simulink model "Controllori"  (R2020b)
settings: Solver=VariableStepAuto  StartTime=0.0  StopTime=6  RelTol=1e-3
values from neighbouring files (symbols this model uses):
  A_num = eval(A)    [eq_non_linear.m]
  B_num = eval(B)    [eq_non_linear.m]
  C_num = eval(C)    [eq_non_linear.m]
  D_num = eval(D)    [eq_non_linear.m]
  G0_fb_lqr_R = dcgain(reg_fb_lqr_R)    [controlloLQR.m]    (also in lqr_params.m)
  G0_fb_lqr_Y = dcgain(reg_fb_lqr_Y)    [controlloLQR.m]    (also in lqr_params.m)
  G0_fb_lqr_z = dcgain(reg_fb_lqr_z)    [controlloLQR.m]    (also in lqr_params.m)
  G0_fb_R = dcgain(reg_fb_R)    [controllo.m]
  G0_fb_Y = dcgain(reg_fb_Y)    [controllo.m]
  G0_fb_z = dcgain(reg_fb_z)    [controllo.m]
  reg_dir_lqr_R = ss(A_R-B_R*K_lqr_R-L_lqr_R*C_R,L_lqr_R,K_lqr_R,0)    [controlloLQR.m]    (also in lqr_params.m)
  reg_dir_lqr_Y = ss(A_Y-B_Y*K_lqr_Y-L_lqr_Y*C_Y,L_lqr_Y,K_lqr_Y,0)    [controlloLQR.m]    (also in lqr_params.m)
  reg_dir_lqr_z = ss(A_z-B_z*K_lqr_z-L_lqr_z*C_z,L_lqr_z,K_lqr_z,0)    [controlloLQR.m]    (also in lqr_params.m)
  reg_dir_R = ss(A_R-B_R*K_R-L_R*C_R,L_R,K_R,0)    [controllo.m]
  reg_dir_Y = ss(A_Y-B_Y*K_Y-L_Y*C_Y,L_Y,K_Y,0)    [controllo.m]
  reg_dir_z = ss(A_z-B_z*K_z-L_z*C_z,L_z,K_z,0)    [controllo.m]
  reg_fb_lqr_R = ss(A_R-B_R*K_lqr_R-L_lqr_R*C_R,-L_lqr_R,-K_lqr_R,0)    [controlloLQR.m]    (also in lqr_params.m)
  reg_fb_lqr_Y = ss(A_Y-B_Y*K_lqr_Y-L_lqr_Y*C_Y,-L_lqr_Y,-K_lqr_Y,0)    [controlloLQR.m]    (also in lqr_params.m)
  reg_fb_lqr_z = ss(A_z-B_z*K_lqr_z-L_lqr_z*C_z,-L_lqr_z,-K_lqr_z,0)    [controlloLQR.m]    (also in lqr_params.m)
  reg_fb_R = ss(A_R-B_R*K_R-L_R*C_R,-L_R,-K_R,0)    [controllo.m]
  reg_fb_Y = ss(A_Y-B_Y*K_Y-L_Y*C_Y,-L_Y,-K_Y,0)    [controllo.m]
  reg_fb_z = ss(A_z-B_z*K_z-L_z*C_z,-L_z,-K_z,0)    [controllo.m]
undefined symbols (not defined in the file or in its folder): A_PID, B_PID, C_PID, D_PID
libraries: pid_lib x8, simulink x1
settings Model: Creator=Tommaso  LastModifiedBy=Tommaso

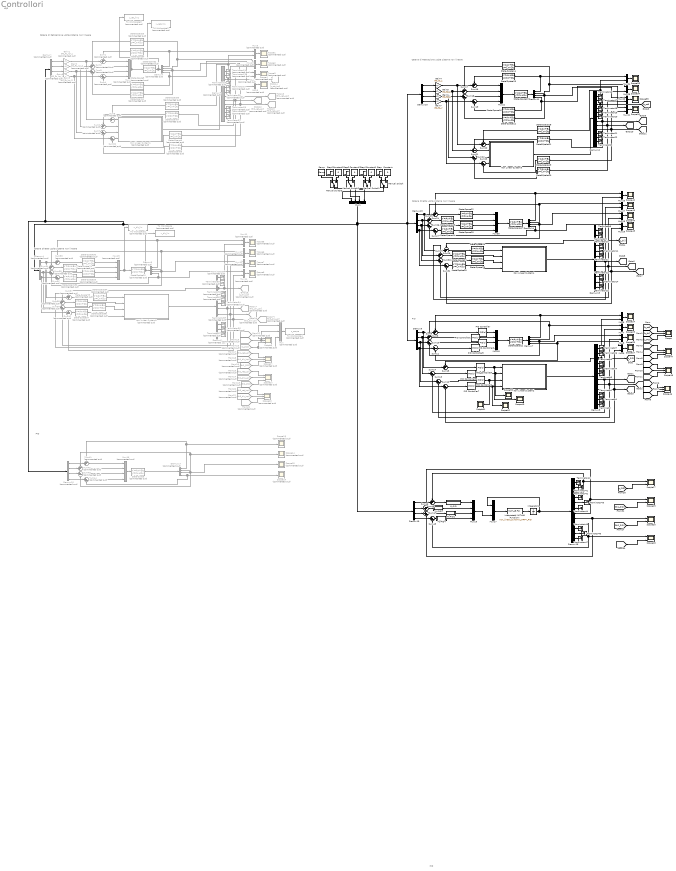
== system Controllori ==
  note: PID
  note: LQR
  note: PID
  note: Catena di Retroazione uscite sistema non lineare
  note: Catena Diretta uscita sistema non lineare
  note: Catena di Retroazione uscite sistema non lineare
  note: Catena Diretta uscita sistema non lineare
  note: PID
  Constant{,1..3} (4 alike) : Constant  Value=0
  Demux{1..2,4..5,16..17} (6 alike) : Demux  Commented=on
  Demux{7,9..11,13..14,19} (7 alike) : Demux
  Demux{8,12,15,18} (4 alike) : Demux  Outputs=12
  Demux3 : Demux  Commented=on  Outputs=12
  Demux6 : Demux  Commented=on  Outputs=12
  From12 : From  Commented=on  GotoTag=z_ret_Lqr
  From13 : From  Commented=on  GotoTag=z_dir_Lqr
  From14 : From  Commented=on  GotoTag=th2_dir_Lqr
  From15 : From  Commented=on  GotoTag=th2_PID
  From16 : From  Commented=on  GotoTag=z_PID
  From17 : From  Commented=on  GotoTag=th1_ret_Lqr
  From18 : From  Commented=on  GotoTag=th1_dir_Lqr
  From19 : From  Commented=on  GotoTag=th1_PID
  From20 : From  Commented=on  GotoTag=th3_ret_Lqr
  From21 : From  Commented=on  GotoTag=th3_dir_Lqr
  From22 : From  Commented=on  GotoTag=th3_PID
  From23 : From  Commented=on  GotoTag=th2_ret_Lqr
  Gain1 : Gain  Commented=on  Gain=G0_fb_lqr_z
  Gain2 : Gain  Commented=on  Gain=G0_fb_lqr_R
  Gain3 : Gain  Commented=on  Gain=G0_fb_lqr_R
  Gain4 : Gain  Gain=G0_fb_z
  Gain5 : Gain  Gain=G0_fb_R
  Gain6 : Gain  Gain=G0_fb_R
  Gain7 : Gain  Gain=G0_fb_Y
  Gain8 : Gain  Commented=on  Gain=G0_fb_lqr_Y
  Goto12 : Goto  Commented=on  GotoTag=th2_ret_Lqr
  Goto13 : Goto  Commented=on  GotoTag=th3_ret_Lqr
  Goto14 : Goto  Commented=on  GotoTag=z_ret_Lqr
  Goto15 : Goto  Commented=on  GotoTag=th1_ret_Lqr
  Goto16 : Goto  Commented=on  GotoTag=z_dir_Lqr
  Goto17 : Goto  Commented=on  GotoTag=th1_dir_Lqr
  Goto18 : Goto  Commented=on  GotoTag=th2_dir_Lqr
  Goto19 : Goto  Commented=on  GotoTag=th3_dir_Lqr
  Integrator1 : Integrator  InitialCondition=[0,0,0,0,0,0,0,0,0,0,0,0]
  Interpreted MATLAB Function1 : MATLABFcn  MATLABFcn=non_linear_dynamic_HRPY_PID
  Manual Switch{,1..3} (4 alike) : ManualSwitch
  Mux : Mux  Commented=on  Inputs=3
  Mux{1,18..19,22,30} (5 alike) : Mux
  Mux{2..3,5,10..14} (8 alike) : Mux  Commented=on  Inputs=2
  Mux15 : Mux  Commented=on
  Mux16 : Mux  Commented=on
  Mux{6..9,17,20..21,24..29} (13 alike) : Mux  Inputs=2
  Mux4 : Mux  Commented=on
  MyPID : Subsystem
  MyPID1 : Subsystem
  MyPID2 : Subsystem
  MyPID4 : Subsystem
  Non Linear System1 : Subsystem  Commented=on
  Non Linear System2 : Subsystem
  Non Linear System3 : Subsystem
  Non Linear System4 : Subsystem
  Non Linear System5 : Subsystem  Commented=on
  PID Controller : pid_lib/PID Controller  Controller=PID  Form=Parallel  TimeDomain=Continuous-time  UseExternalTs=off  SampleTime=-1  IntegratorMethod=Forward Euler  FilterMethod=Forward Euler  ControllerParametersSource=internal  P=10  I=6  D=10  UseFilter=on  N=100  TunerSelectOption=Transfer Function Based (PID Tuner App)  InitialConditionSource=internal  InitialConditionForIntegrator=0  InitialConditionForFilter=0  DifferentiatorICPrevScaledInput=0  ExternalReset=none  TrackingMode=off  Kt=1  LimitOutput=off  SatLimitsSource=internal  UpperSaturationLimit=40  LowerSaturationLimit=-40  LinearizeAsGain=on  AntiWindupMode=none  Kb=1  POutMin=[]  POutMax=[]  IOutMin=[]  IOutMax=[]  DOutMin=[]  DOutMax=[]  NOutMin=[]  NOutMax=[]  SumOutMin=[]  SumOutMax=[]  SaturationOutMin=[]  SaturationOutMax=[]  PParamMin=[]  PParamMax=[]  IParamMin=[]  IParamMax=[]  DParamMin=[]  DParamMax=[]  NParamMin=[]  NParamMax=[]  KbParamMin=[]  KbParamMax=[]  KtParamMin=[]  KtParamMax=[]  KbOutMin=[]  KbOutMax=[]  KtOutMin=[]  KtOutMax=[]  IntegratorOutMin=[]  IntegratorOutMax=[]  FilterOutMin=[]  FilterOutMax=[]  SumI1OutMin=[]  SumI1OutMax=[]  SumI2OutMin=[]  SumI2OutMax=[]  SumI3OutMin=[]  SumI3OutMax=[]  SumI4OutMin=[]  SumI4OutMax=[]  SumDOutMin=[]  SumDOutMax=[]  DifferentiatorOutMin=[]  DifferentiatorOutMax=[]  FilterDiffOutCoefMin=[]  FilterDiffOutCoefMax=[]  ReciprocalOutMin=[]  ReciprocalOutMax=[]  SumDenOutMin=[]  SumDenOutMax=[]  SumNumOutMin=[]  SumNumOutMax=[]  DivideOutMin=[]  DivideOutMax=[]  UdiffTsProdOutMin=[]  UdiffTsProdOutMax=[]  NTsProdOutMin=[]  NTsProdOutMax=[]  UintegralTsProdOutMin=[]  UintegralTsProdOutMax=[]  UngainTsProdOutMin=[]  UngainTsProdOutMax=[]  IntegratorContinuousStateAttributes=''  IntegratorStateMustResolveToSignalObject=off  IntegratorRTWStateStorageClass=Auto  FilterContinuousStateAttributes=''  FilterStateMustResolveToSignalObject=off  FilterRTWStateStorageClass=Auto  ParallelPVariant=InternalParameters  IdealPVariant=Disabled  IVariant=InternalParameters  DVariant=InternalParameters  IntegratorVariant=Continuous  SatVariant=Disabled  AWVariant=Passthrough  PCopyVariant=Disabled  TRVariant=Disabled  FdbkBlocksVariant=Forward  IdealPFdbkVariant=Disabled  SatFdbkVariant=Disabled  DerivativeFilterVariant=ContFilter  NVariant=InternalParameters  NCopyVariant=Disabled  FilterICVariant=InternalICsFilter  IntegratorICVariant=InternalICs  ExternalResetVariant=Disabled  TRSumVariant=Passthrough  SumFdbkVariant=Disabled  SumVariant=Sum_PID  TsampFilterVariant=InternalTs  TsampNgainVariant=Passthrough  TsampIntegralVariant=Passthrough  ExternalSaturationOutDataTypeStr=Inherit: Same as second input
  PID Controller{1..2,5..6} (4 alike) : pid_lib/PID Controller  Controller=PID  Form=Parallel  TimeDomain=Continuous-time  UseExternalTs=off  SampleTime=-1  IntegratorMethod=Forward Euler  FilterMethod=Forward Euler  ControllerParametersSource=internal  P=1  I=1  D=0.5  UseFilter=on  N=100  TunerSelectOption=Transfer Function Based (PID Tuner App)  InitialConditionSource=internal  InitialConditionForIntegrator=0  InitialConditionForFilter=0  DifferentiatorICPrevScaledInput=0  ExternalReset=none  TrackingMode=off  Kt=1  LimitOutput=off  SatLimitsSource=internal  UpperSaturationLimit=inf  LowerSaturationLimit=-inf  LinearizeAsGain=on  AntiWindupMode=none  Kb=1  POutMin=[]  POutMax=[]  IOutMin=[]  IOutMax=[]  DOutMin=[]  DOutMax=[]  NOutMin=[]  NOutMax=[]  SumOutMin=[]  SumOutMax=[]  SaturationOutMin=[]  SaturationOutMax=[]  PParamMin=[]  PParamMax=[]  IParamMin=[]  IParamMax=[]  DParamMin=[]  DParamMax=[]  NParamMin=[]  NParamMax=[]  KbParamMin=[]  KbParamMax=[]  KtParamMin=[]  KtParamMax=[]  KbOutMin=[]  KbOutMax=[]  KtOutMin=[]  KtOutMax=[]  IntegratorOutMin=[]  IntegratorOutMax=[]  FilterOutMin=[]  FilterOutMax=[]  SumI1OutMin=[]  SumI1OutMax=[]  SumI2OutMin=[]  SumI2OutMax=[]  SumI3OutMin=[]  SumI3OutMax=[]  SumI4OutMin=[]  SumI4OutMax=[]  SumDOutMin=[]  SumDOutMax=[]  DifferentiatorOutMin=[]  DifferentiatorOutMax=[]  FilterDiffOutCoefMin=[]  FilterDiffOutCoefMax=[]  ReciprocalOutMin=[]  ReciprocalOutMax=[]  SumDenOutMin=[]  SumDenOutMax=[]  SumNumOutMin=[]  SumNumOutMax=[]  DivideOutMin=[]  DivideOutMax=[]  UdiffTsProdOutMin=[]  UdiffTsProdOutMax=[]  NTsProdOutMin=[]  NTsProdOutMax=[]  UintegralTsProdOutMin=[]  UintegralTsProdOutMax=[]  UngainTsProdOutMin=[]  UngainTsProdOutMax=[]  IntegratorContinuousStateAttributes=''  IntegratorStateMustResolveToSignalObject=off  IntegratorRTWStateStorageClass=Auto  FilterContinuousStateAttributes=''  FilterStateMustResolveToSignalObject=off  FilterRTWStateStorageClass=Auto  ParallelPVariant=InternalParameters  IdealPVariant=Disabled  IVariant=InternalParameters  DVariant=InternalParameters  IntegratorVariant=Continuous  SatVariant=Disabled  AWVariant=Passthrough  PCopyVariant=Disabled  TRVariant=Disabled  FdbkBlocksVariant=Forward  IdealPFdbkVariant=Disabled  SatFdbkVariant=Disabled  DerivativeFilterVariant=ContFilter  NVariant=InternalParameters  NCopyVariant=Disabled  FilterICVariant=InternalICsFilter  IntegratorICVariant=InternalICs  ExternalResetVariant=Disabled  TRSumVariant=Passthrough  SumFdbkVariant=Disabled  SumVariant=Sum_PID  TsampFilterVariant=InternalTs  TsampNgainVariant=Passthrough  TsampIntegralVariant=Passthrough  ExternalSaturationOutDataTypeStr=Inherit: Same as second input
  PID Controller3 : pid_lib/PID Controller  Controller=PID  Form=Parallel  TimeDomain=Continuous-time  UseExternalTs=off  SampleTime=-1  IntegratorMethod=Forward Euler  FilterMethod=Forward Euler  ControllerParametersSource=internal  P=1  I=1  D=1  UseFilter=on  N=100  TunerSelectOption=Transfer Function Based (PID Tuner App)  InitialConditionSource=internal  InitialConditionForIntegrator=0  InitialConditionForFilter=0  DifferentiatorICPrevScaledInput=0  ExternalReset=none  TrackingMode=off  Kt=1  LimitOutput=off  SatLimitsSource=internal  UpperSaturationLimit=inf  LowerSaturationLimit=-inf  LinearizeAsGain=on  AntiWindupMode=none  Kb=1  POutMin=[]  POutMax=[]  IOutMin=[]  IOutMax=[]  DOutMin=[]  DOutMax=[]  NOutMin=[]  NOutMax=[]  SumOutMin=[]  SumOutMax=[]  SaturationOutMin=[]  SaturationOutMax=[]  PParamMin=[]  PParamMax=[]  IParamMin=[]  IParamMax=[]  DParamMin=[]  DParamMax=[]  NParamMin=[]  NParamMax=[]  KbParamMin=[]  KbParamMax=[]  KtParamMin=[]  KtParamMax=[]  KbOutMin=[]  KbOutMax=[]  KtOutMin=[]  KtOutMax=[]  IntegratorOutMin=[]  IntegratorOutMax=[]  FilterOutMin=[]  FilterOutMax=[]  SumI1OutMin=[]  SumI1OutMax=[]  SumI2OutMin=[]  SumI2OutMax=[]  SumI3OutMin=[]  SumI3OutMax=[]  SumI4OutMin=[]  SumI4OutMax=[]  SumDOutMin=[]  SumDOutMax=[]  DifferentiatorOutMin=[]  DifferentiatorOutMax=[]  FilterDiffOutCoefMin=[]  FilterDiffOutCoefMax=[]  ReciprocalOutMin=[]  ReciprocalOutMax=[]  SumDenOutMin=[]  SumDenOutMax=[]  SumNumOutMin=[]  SumNumOutMax=[]  DivideOutMin=[]  DivideOutMax=[]  UdiffTsProdOutMin=[]  UdiffTsProdOutMax=[]  NTsProdOutMin=[]  NTsProdOutMax=[]  UintegralTsProdOutMin=[]  UintegralTsProdOutMax=[]  UngainTsProdOutMin=[]  UngainTsProdOutMax=[]  IntegratorContinuousStateAttributes=''  IntegratorStateMustResolveToSignalObject=off  IntegratorRTWStateStorageClass=Auto  FilterContinuousStateAttributes=''  FilterStateMustResolveToSignalObject=off  FilterRTWStateStorageClass=Auto  ParallelPVariant=InternalParameters  IdealPVariant=Disabled  IVariant=InternalParameters  DVariant=InternalParameters  IntegratorVariant=Continuous  SatVariant=Disabled  AWVariant=Passthrough  PCopyVariant=Disabled  TRVariant=Disabled  FdbkBlocksVariant=Forward  IdealPFdbkVariant=Disabled  SatFdbkVariant=Disabled  DerivativeFilterVariant=ContFilter  NVariant=InternalParameters  NCopyVariant=Disabled  FilterICVariant=InternalICsFilter  IntegratorICVariant=InternalICs  ExternalResetVariant=Disabled  TRSumVariant=Passthrough  SumFdbkVariant=Disabled  SumVariant=Sum_PID  TsampFilterVariant=InternalTs  TsampNgainVariant=Passthrough  TsampIntegralVariant=Passthrough  ExternalSaturationOutDataTypeStr=Inherit: Same as second input
  PID Controller4 : pid_lib/PID Controller  Controller=PID  Form=Parallel  TimeDomain=Continuous-time  UseExternalTs=off  SampleTime=-1  IntegratorMethod=Forward Euler  FilterMethod=Forward Euler  ControllerParametersSource=internal  P=10  I=6  D=10  UseFilter=on  N=100  TunerSelectOption=Transfer Function Based (PID Tuner App)  InitialConditionSource=internal  InitialConditionForIntegrator=0  InitialConditionForFilter=0  DifferentiatorICPrevScaledInput=0  ExternalReset=none  TrackingMode=off  Kt=1  LimitOutput=off  SatLimitsSource=internal  UpperSaturationLimit=40  LowerSaturationLimit=-40  LinearizeAsGain=on  AntiWindupMode=none  Kb=1  POutMin=[]  POutMax=[]  IOutMin=[]  IOutMax=[]  DOutMin=[]  DOutMax=[]  NOutMin=[]  NOutMax=[]  SumOutMin=[]  SumOutMax=[]  SaturationOutMin=[]  SaturationOutMax=[]  PParamMin=[]  PParamMax=[]  IParamMin=[]  IParamMax=[]  DParamMin=[]  DParamMax=[]  NParamMin=[]  NParamMax=[]  KbParamMin=[]  KbParamMax=[]  KtParamMin=[]  KtParamMax=[]  KbOutMin=[]  KbOutMax=[]  KtOutMin=[]  KtOutMax=[]  IntegratorOutMin=[]  IntegratorOutMax=[]  FilterOutMin=[]  FilterOutMax=[]  SumI1OutMin=[]  SumI1OutMax=[]  SumI2OutMin=[]  SumI2OutMax=[]  SumI3OutMin=[]  SumI3OutMax=[]  SumI4OutMin=[]  SumI4OutMax=[]  SumDOutMin=[]  SumDOutMax=[]  DifferentiatorOutMin=[]  DifferentiatorOutMax=[]  FilterDiffOutCoefMin=[]  FilterDiffOutCoefMax=[]  ReciprocalOutMin=[]  ReciprocalOutMax=[]  SumDenOutMin=[]  SumDenOutMax=[]  SumNumOutMin=[]  SumNumOutMax=[]  DivideOutMin=[]  DivideOutMax=[]  UdiffTsProdOutMin=[]  UdiffTsProdOutMax=[]  NTsProdOutMin=[]  NTsProdOutMax=[]  UintegralTsProdOutMin=[]  UintegralTsProdOutMax=[]  UngainTsProdOutMin=[]  UngainTsProdOutMax=[]  IntegratorContinuousStateAttributes=''  IntegratorStateMustResolveToSignalObject=off  IntegratorRTWStateStorageClass=Auto  FilterContinuousStateAttributes=''  FilterStateMustResolveToSignalObject=off  FilterRTWStateStorageClass=Auto  ParallelPVariant=InternalParameters  IdealPVariant=Disabled  IVariant=InternalParameters  DVariant=InternalParameters  IntegratorVariant=Continuous  SatVariant=Disabled  AWVariant=Passthrough  PCopyVariant=Disabled  TRVariant=Disabled  FdbkBlocksVariant=Forward  IdealPFdbkVariant=Disabled  SatFdbkVariant=Disabled  DerivativeFilterVariant=ContFilter  NVariant=InternalParameters  NCopyVariant=Disabled  FilterICVariant=InternalICsFilter  IntegratorICVariant=InternalICs  ExternalResetVariant=Disabled  TRSumVariant=Passthrough  SumFdbkVariant=Disabled  SumVariant=Sum_PID  TsampFilterVariant=InternalTs  TsampNgainVariant=Passthrough  TsampIntegralVariant=Passthrough  ExternalSaturationOutDataTypeStr=Inherit: Same as second input
  PID Controller7 : pid_lib/PID Controller  Controller=PID  Form=Parallel  TimeDomain=Continuous-time  UseExternalTs=off  SampleTime=-1  IntegratorMethod=Forward Euler  FilterMethod=Forward Euler  ControllerParametersSource=internal  P=1  I=1  D=1  UseFilter=on  N=100  TunerSelectOption=Transfer Function Based (PID Tuner App)  InitialConditionSource=internal  InitialConditionForIntegrator=0  InitialConditionForFilter=0  DifferentiatorICPrevScaledInput=0  ExternalReset=none  TrackingMode=off  Kt=1  LimitOutput=off  SatLimitsSource=internal  UpperSaturationLimit=inf  LowerSaturationLimit=-inf  LinearizeAsGain=on  AntiWindupMode=none  Kb=1  POutMin=[]  POutMax=[]  IOutMin=[]  IOutMax=[]  DOutMin=[]  DOutMax=[]  NOutMin=[]  NOutMax=[]  SumOutMin=[]  SumOutMax=[]  SaturationOutMin=[]  SaturationOutMax=[]  PParamMin=[]  PParamMax=[]  IParamMin=[]  IParamMax=[]  DParamMin=[]  DParamMax=[]  NParamMin=[]  NParamMax=[]  KbParamMin=[]  KbParamMax=[]  KtParamMin=[]  KtParamMax=[]  KbOutMin=[]  KbOutMax=[]  KtOutMin=[]  KtOutMax=[]  IntegratorOutMin=[]  IntegratorOutMax=[]  FilterOutMin=[]  FilterOutMax=[]  SumI1OutMin=[]  SumI1OutMax=[]  SumI2OutMin=[]  SumI2OutMax=[]  SumI3OutMin=[]  SumI3OutMax=[]  SumI4OutMin=[]  SumI4OutMax=[]  SumDOutMin=[]  SumDOutMax=[]  DifferentiatorOutMin=[]  DifferentiatorOutMax=[]  FilterDiffOutCoefMin=[]  FilterDiffOutCoefMax=[]  ReciprocalOutMin=[]  ReciprocalOutMax=[]  SumDenOutMin=[]  SumDenOutMax=[]  SumNumOutMin=[]  SumNumOutMax=[]  DivideOutMin=[]  DivideOutMax=[]  UdiffTsProdOutMin=[]  UdiffTsProdOutMax=[]  NTsProdOutMin=[]  NTsProdOutMax=[]  UintegralTsProdOutMin=[]  UintegralTsProdOutMax=[]  UngainTsProdOutMin=[]  UngainTsProdOutMax=[]  IntegratorContinuousStateAttributes=''  IntegratorStateMustResolveToSignalObject=off  IntegratorRTWStateStorageClass=Auto  FilterContinuousStateAttributes=''  FilterStateMustResolveToSignalObject=off  FilterRTWStateStorageClass=Auto  ParallelPVariant=InternalParameters  IdealPVariant=Disabled  IVariant=InternalParameters  DVariant=InternalParameters  IntegratorVariant=Continuous  SatVariant=Disabled  AWVariant=Passthrough  PCopyVariant=Disabled  TRVariant=Disabled  FdbkBlocksVariant=Forward  IdealPFdbkVariant=Disabled  SatFdbkVariant=Disabled  DerivativeFilterVariant=ContFilter  NVariant=InternalParameters  NCopyVariant=Disabled  FilterICVariant=InternalICsFilter  IntegratorICVariant=InternalICs  ExternalResetVariant=Disabled  TRSumVariant=Passthrough  SumFdbkVariant=Disabled  SumVariant=Sum_PID  TsampFilterVariant=InternalTs  TsampNgainVariant=Passthrough  TsampIntegralVariant=Passthrough  ExternalSaturationOutDataTypeStr=Inherit: Same as second input
  Ramp : simulink/Sources/Ramp  slope=0.2  start=1  InitialOutput=0
  Scope{,46..48} (4 alike) : Scope  NumInputPorts=3
  Scope{1..8,13..16} (12 alike) : Scope  Commented=on
  Scope{9..12} (4 alike) : Scope  Commented=on  NumInputPorts=3
  Scope{17..20} (4 alike) : Scope  NumInputPorts=2
  Scope{24..27,33..36,42..45,49..52} (16 alike) : Scope
  State-Space : StateSpace  Commented=on  A=A_PID  B=B_PID  C=C_PID  D=D_PID  InitialCondition=0
  State-Space{1,3,7..8} (4 alike) : StateSpace  Commented=on  A=reg_fb_lqr_R.a  B=reg_fb_lqr_R.b  C=reg_fb_lqr_R.c  D=reg_fb_lqr_R.d  InitialCondition=0
  State-Space10 : StateSpace  Commented=on  A=A_num  B=B_num  C=C_num  D=D_num  InitialCondition=0
  State-Space11 : StateSpace  A=A_num  B=B_num  C=C_num  D=D_num  InitialCondition=0
  State-Space{12,14,20..21} (4 alike) : StateSpace  A=reg_fb_R.a  B=reg_fb_R.b  C=reg_fb_R.c  D=reg_fb_R.d  InitialCondition=0
  State-Space13 : StateSpace  A=A_num  B=B_num  C=C_num  D=D_num  InitialCondition=0
  State-Space15 : StateSpace  A=reg_fb_z.a  B=reg_fb_z.b  C=reg_fb_z.c  D=reg_fb_z.d  InitialCondition=0
  State-Space16 : StateSpace  A=reg_fb_Y.a  B=reg_fb_Y.b  C=reg_fb_Y.c  D=reg_fb_Y.d  InitialCondition=0
  State-Space17 : StateSpace  A=A_num  B=B_num  C=C_num  D=D_num  InitialCondition=0
  State-Space18 : StateSpace  A=reg_fb_z.a  B=reg_fb_z.b  C=reg_fb_z.c  D=reg_fb_z.d  InitialCondition=0
  State-Space19 : StateSpace  A=reg_fb_Y.a  B=reg_fb_Y.b  C=reg_fb_Y.c  D=reg_fb_Y.d  InitialCondition=0
  State-Space2 : StateSpace  Commented=on  A=A_num  B=B_num  C=C_num  D=D_num  InitialCondition=0
  State-Space22 : StateSpace  A=reg_dir_z.a  B=reg_dir_z.b  C=reg_dir_z.c  D=reg_dir_z.d  InitialCondition=0
  State-Space{23,25,27,29} (4 alike) : StateSpace  A=reg_dir_R.a  B=reg_dir_R.b  C=reg_dir_R.c  D=reg_dir_R.d  InitialCondition=0
  State-Space24 : StateSpace  A=reg_dir_Y.a  B=reg_dir_Y.b  C=reg_dir_Y.c  D=reg_dir_Y.d  InitialCondition=0
  State-Space26 : StateSpace  A=reg_dir_z.a  B=reg_dir_z.b  C=reg_dir_z.c  D=reg_dir_z.d  InitialCondition=0
  State-Space28 : StateSpace  A=reg_dir_Y.a  B=reg_dir_Y.b  C=reg_dir_Y.c  D=reg_dir_Y.d  InitialCondition=0
  State-Space30 : StateSpace  Commented=on  A=reg_dir_lqr_z.a  B=reg_dir_lqr_z.b  C=reg_dir_lqr_z.c  D=reg_dir_lqr_z.d  InitialCondition=0
  State-Space{31,33,35..36} (4 alike) : StateSpace  Commented=on  A=reg_dir_lqr_R.a  B=reg_dir_lqr_R.b  C=reg_dir_lqr_R.c  D=reg_dir_lqr_R.d  InitialCondition=0
  State-Space32 : StateSpace  Commented=on  A=reg_dir_lqr_Y.a  B=reg_dir_lqr_Y.b  C=reg_dir_lqr_Y.c  D=reg_dir_lqr_Y.d  InitialCondition=0
  State-Space34 : StateSpace  Commented=on  A=reg_dir_lqr_z.a  B=reg_dir_lqr_z.b  C=reg_dir_lqr_z.c  D=reg_dir_lqr_z.d  InitialCondition=0
  State-Space37 : StateSpace  Commented=on  A=reg_dir_lqr_Y.a  B=reg_dir_lqr_Y.b  C=reg_dir_lqr_Y.c  D=reg_dir_lqr_Y.d  InitialCondition=0
  State-Space4 : StateSpace  Commented=on  A=reg_fb_lqr_z.a  B=reg_fb_lqr_z.b  C=reg_fb_lqr_z.c  D=reg_fb_lqr_z.d  InitialCondition=0
  State-Space5 : StateSpace  Commented=on  A=reg_fb_lqr_Y.a  B=reg_fb_lqr_Y.b  C=reg_fb_lqr_Y.c  D=reg_fb_lqr_Y.d  InitialCondition=0
  State-Space6 : StateSpace  Commented=on  A=reg_fb_lqr_z.a  B=reg_fb_lqr_z.b  C=reg_fb_lqr_z.c  D=reg_fb_lqr_z.d  InitialCondition=0
  State-Space9 : StateSpace  Commented=on  A=reg_fb_lqr_Y.a  B=reg_fb_lqr_Y.b  C=reg_fb_lqr_Y.c  D=reg_fb_lqr_Y.d  InitialCondition=0
  Step : Step  SampleTime=0
  Step1 : Step  After=0.3  SampleTime=0
  Step2 : Step  After=0.3  SampleTime=0
  Step3 : Step  After=0.1  SampleTime=0
  Sum{1..2,5..6,33..34,37..38,41..42} (10 alike) : Sum  Commented=on  Inputs=-+|
  Sum{10..14,18..19,22..23,26..27,30..31,47..48} (15 alike) : Sum  Inputs=|+-
  Sum{8..9,15..17,20..21,24..25,28..29,45..46} (13 alike) : Sum  Inputs=-+|
  Sum{3..4,7,32,35..36,39..40,43..44} (10 alike) : Sum  Commented=on  Inputs=|+-
  Terminator{,1..23,40..47} (32 alike) : Terminator
  Terminator{24..39} (16 alike) : Terminator  Commented=on
  To Workspace : ToWorkspace  Commented=on  VariableName=x_dir_lin  SaveFormat=Timeseries  SampleTime=-1
  To Workspace1 : ToWorkspace  Commented=on  VariableName=u_dir_lin  SaveFormat=Timeseries  SampleTime=-1
  To Workspace2 : ToWorkspace  Commented=on  VariableName=x_ret_lin1  SaveFormat=Timeseries  SampleTime=-1
  To Workspace3 : ToWorkspace  Commented=on  VariableName=u_ret_lin1  SaveFormat=Timeseries  SampleTime=-1
  To Workspace4 : ToWorkspace  Commented=on  VariableName=z_scope  SaveFormat=Timeseries  SampleTime=-1
  wires:
  Manual Switch3/1 -> Mux1/4
  Manual Switch1/1 -> Mux1/2
  Manual Switch2/1 -> Mux1/3
  Manual Switch/1 -> Mux1/1
  PID Controller/1 -> Mux18/1
  Mux7/1 -> Scope25/1
  Demux9/1 -> Sum15/2, Sum8/2
  PID Controller2/1 -> Mux18/3
  Demux9/2 -> Sum14/1, Sum9/2
  PID Controller3/1 -> Mux18/4
  Demux7/4 -> Sum11/2, Mux9/1  "\\theta_3_lin"
  Sum11/1 -> PID Controller3/1
  Demux7/2 -> Mux7/1, Sum9/1  "\\theta_1_lin"
  Sum9/1 -> PID Controller1/1
  Demux8/8 -> [th2_PID], Mux8/2, Sum13/2  "\\theta_2"
  Demux7/3 -> Sum10/2, Mux8/1  "\\theta_2_lin"
  Sum10/1 -> PID Controller2/1
  Sum8/1 -> PID Controller/1
  Demux8/9 -> [th3_PID], Mux9/2, Sum12/2  "\\theta_3"
  Mux6/1 -> Scope24/1
  Mux8/1 -> Scope26/1
  Demux9/3 -> Sum13/1, Sum10/1
  Demux8/3 -> [z_PID], Mux6/2, Sum15/1  "z"
  State-Space11/1 -> Demux7/1
  PID Controller1/1 -> Mux18/2
  Non Linear System2/1(y) -> Demux8/1
  Mux18/1 -> State-Space11/1
  Demux7/1 -> Sum8/1, Mux6/1  "z_lin"
  Demux8/7 -> [th1_PID], Sum14/2, Mux7/2  "\\theta_1"
  Mux9/1 -> Scope27/1
  Demux9/4 -> Sum12/1, Sum11/1
  PID Controller4/1 -> Scope49/1, Non Linear System2/1(H)
  PID Controller5/1 -> Scope50/1, Non Linear System2/2(R)
  PID Controller6/1 -> Non Linear System2/3(P), Scope51/1
  PID Controller7/1 -> Non Linear System2/4(Y), Scope52/1
  Sum12/1 -> PID Controller7/1
  Sum14/1 -> PID Controller5/1
  Sum15/1 -> PID Controller4/1
  Sum13/1 -> PID Controller6/1
  Non Linear System3/1(y) -> Demux12/1
  Gain6/1 -> Sum18/1, Sum22/1
  Gain5/1 -> Sum21/2, Sum17/2
  Demux10/1 -> Gain4/1
  Demux10/2 -> Gain5/1
  Gain7/1 -> Sum23/1, Sum19/1
  Mux20/1 -> Scope35/1
  State-Space13/1 -> Demux11/1
  Mux22/1 -> State-Space13/1
  Demux11/2 -> State-Space14/1, Mux25/1  "\\theta_1_lin"
  Demux11/3 -> State-Space12/1, Mux20/1  "\\theta_2_lin"
  State-Space14/1 -> Sum17/1
  State-Space16/1 -> Sum19/2
  Mux24/1 -> Scope33/1
  Gain4/1 -> Sum20/2, Sum16/2
  Sum16/1 -> Mux22/1
  Demux12/9 -> State-Space19/1, [th3_ret], Mux21/2  "\\theta_3"
  Demux11/1 -> State-Space15/1, Mux24/1  "z_lin"
  Demux12/7 -> State-Space21/1, [th1_ret], Mux25/2  "\\theta_1"
  Demux12/3 -> [z_ret], Mux24/2, State-Space18/1  "z"
  State-Space12/1 -> Sum18/2
  Mux21/1 -> Scope36/1
  Demux11/4 -> Mux21/1, State-Space16/1  "\\theta_3_lin"
  Sum19/1 -> Mux22/4
  Sum17/1 -> Mux22/2
  Sum18/1 -> Mux22/3
  Mux25/1 -> Scope34/1
  State-Space15/1 -> Sum16/1
  Demux10/3 -> Gain6/1
  Demux10/4 -> Gain7/1
  Sum21/1 -> Non Linear System3/2(R)
  Sum20/1 -> Non Linear System3/1(H)
  Sum22/1 -> Non Linear System3/3(P)
  Sum23/1 -> Non Linear System3/4(Y)
  State-Space18/1 -> Sum20/1
  State-Space21/1 -> Sum21/1
  State-Space19/1 -> Sum23/2
  State-Space20/1 -> Sum22/2
  State-Space17/1 -> Demux14/1
  Demux14/4 -> Mux29/1, Sum27/2  "\\theta_3_lin"
  Mux28/1 -> Scope44/1
  Sum26/1 -> State-Space25/1
  State-Space23/1 -> Mux30/2
  Demux14/3 -> Sum26/2, Mux28/1  "\\theta_2_lin"
  Demux14/2 -> Mux27/1, Sum25/1  "\\theta_1_lin"
  Mux30/1 -> State-Space17/1
  Mux26/1 -> Scope42/1
  Demux15/7 -> Mux27/2, [th1_dri], Sum29/1  "\\theta_1"
  Demux15/8 -> [th2_dri], Mux28/2, Sum30/2  "\\theta_2"
  Sum24/1 -> State-Space22/1
  State-Space25/1 -> Mux30/3
  Sum27/1 -> State-Space24/1
  State-Space22/1 -> Mux30/1
  Demux14/1 -> Sum24/1, Mux26/1  "z_lin"
  Non Linear System4/1(y) -> Demux15/1
  Sum25/1 -> State-Space23/1
  Demux15/3 -> [z_dri], Mux26/2, Sum28/1  "z"
  Mux27/1 -> Scope43/1
  Mux29/1 -> Scope45/1
  State-Space24/1 -> Mux30/4
  Sum29/1 -> State-Space27/1
  Demux13/3 -> Sum30/1, Sum26/1
  Demux13/1 -> Sum28/2, Sum24/2
  Sum31/1 -> State-Space28/1
  Demux13/4 -> Sum31/1, Sum27/1
  Demux13/2 -> Sum29/2, Sum25/2
  Sum30/1 -> State-Space29/1
  Sum28/1 -> State-Space26/1
  State-Space28/1 -> Non Linear System4/4(Y)
  State-Space29/1 -> Non Linear System4/3(P)
  State-Space27/1 -> Non Linear System4/2(R)
  State-Space26/1 -> Non Linear System4/1(H)
  Demux8/12 -> Terminator/1
  Demux8/11 -> Terminator1/1
  Demux8/10 -> Terminator2/1
  Demux8/6 -> Terminator3/1
  Demux8/5 -> Terminator4/1
  Demux8/4 -> Terminator5/1
  Demux8/2 -> Terminator6/1  "y"
  Demux8/1 -> Terminator7/1  "x"
  Demux15/1 -> Terminator8/1  "x"
  Demux15/2 -> Terminator9/1  "y"
  Demux15/4 -> Terminator10/1
  Demux15/5 -> Terminator11/1
  Demux15/6 -> Terminator12/1
  Demux15/10 -> Terminator13/1
  Demux15/11 -> Terminator14/1
  Demux15/12 -> Terminator15/1
  Demux12/1 -> Terminator16/1  "x"
  Demux12/2 -> Terminator17/1  "y"
  Demux12/4 -> Terminator18/1
  Demux12/5 -> Terminator19/1
  Demux12/6 -> Terminator20/1
  Demux12/10 -> Terminator21/1
  Demux12/11 -> Terminator22/1
  Demux12/12 -> Terminator23/1
  [z_ret] -> Scope/1
  [z_dri] -> Scope/2
  [z_PID] -> Scope/3
  [th1_PID] -> Scope47/3
  [th1_dri] -> Scope47/2
  [th1_ret] -> Scope47/1
  [th3_dri] -> Scope46/2
  [th3_ret] -> Scope46/1
  [th3_PID] -> Scope46/3
  [th2_dri] -> Scope48/2
  [th2_ret] -> Scope48/1
  [th2_PID] -> Scope48/3
  Demux15/9 -> Sum31/2, [th3_dri], Mux29/2
  Demux12/8 -> Mux20/2, [th2_ret], State-Space20/1  "\\theta_2"
  Step/1 -> Manual Switch/1
  Constant/1 -> Manual Switch/2
  Ramp/1 -> Manual Switch3/1
  Constant3/1 -> Manual Switch3/2
  Step2/1 -> Manual Switch2/1
  Constant2/1 -> Manual Switch2/2
  Step1/1 -> Manual Switch1/1
  Constant1/1 -> Manual Switch1/2
  Sum4/1 -> Mux4/4
  Demux3/7 -> State-Space7/1, Goto15/1, Mux10/2  "\\theta_1"
  State-Space8/1 -> Sum7/2
  Demux2/2 -> State-Space3/1, Mux10/1  "\\theta_1_lin"
  Sum6/1 -> Non Linear System1/2(R)
  State-Space4/1 -> Sum1/1
  State-Space6/1 -> Sum5/1
  Demux3/2 -> Terminator25/1  "y"
  State-Space3/1 -> Sum2/1
  Demux3/4 -> Terminator26/1
  Demux3/6 -> Terminator28/1
  Demux3/5 -> Terminator27/1
  Sum32/1 -> Non Linear System1/4(Y)
  State-Space2/1 -> To Workspace2/1, Demux2/1
  Gain1/1 -> Sum5/2, Sum1/2
  Mux5/1 -> Scope1/1
  State-Space9/1 -> Sum32/2
  State-Space7/1 -> Sum6/1
  Sum3/1 -> Mux4/3
  Demux2/4 -> Mux3/1, State-Space5/1  "\\theta_3_lin"
  Demux3/8 -> State-Space8/1, Mux2/2, Goto12/1  "\\theta_2"
  State-Space1/1 -> Sum3/2
  Mux3/1 -> Scope4/1
  Mux2/1 -> Scope3/1
  Demux3/11 -> Terminator30/1
  Demux3/12 -> Terminator31/1
  Sum2/1 -> Mux4/2
  Mux10/1 -> Scope2/1
  Gain3/1 -> Sum3/1, Sum7/1
  Demux3/9 -> State-Space9/1, Goto13/1, Mux3/2  "\\theta_3"
  Demux3/3 -> Goto14/1, State-Space6/1, Mux5/2  "z"
  Sum7/1 -> Non Linear System1/3(P)
  Demux3/10 -> Terminator29/1
  Sum5/1 -> Non Linear System1/1(H)
  Demux1/3 -> Gain3/1
  Demux3/1 -> Terminator24/1  "x"
  Demux2/1 -> State-Space4/1, Mux5/1  "z_lin"
  Sum1/1 -> Mux4/1
  Gain8/1 -> Sum32/1, Sum4/1
  Non Linear System1/1(y) -> Demux3/1
  Demux1/4 -> Gain8/1
  Gain2/1 -> Sum6/2, Sum2/2
  Demux1/2 -> Gain2/1
  State-Space5/1 -> Sum4/2
  Mux4/1 -> To Workspace3/1, State-Space2/1
  Demux2/3 -> State-Space1/1, Mux2/1  "\\theta_2_lin"
  Demux1/1 -> Gain1/1
  Sum39/1 -> State-Space36/1
  State-Space35/1 -> Non Linear System5/2(R)
  Mux13/1 -> Scope7/1
  Demux6/1 -> Terminator38/1  "x"
  Sum38/1 -> State-Space35/1
  Demux6/8 -> Goto18/1, Mux13/2, Sum39/2  "\\theta_2"
  Sum40/1 -> State-Space37/1
  Demux6/5 -> Terminator33/1
  Demux6/3 -> Goto16/1, Mux11/2, Sum37/1  "z"
  Demux6/6 -> Terminator34/1
  Demux6/4 -> Terminator32/1
  Demux5/1 -> Sum33/1, Mux11/1  "z_lin"
  Demux4/1 -> Sum37/2, Sum33/2
  Demux4/3 -> Sum39/1, Sum35/1
  Mux14/1 -> Scope8/1
  Sum37/1 -> State-Space34/1
  Demux4/2 -> Sum38/2, Sum34/2
  State-Space34/1 -> Non Linear System5/1(H)
  State-Space36/1 -> Non Linear System5/3(P)
  Demux6/11 -> Terminator36/1
  Sum33/1 -> State-Space30/1
  Non Linear System5/1(y) -> Demux6/1
  State-Space33/1 -> Mux15/3
  Mux12/1 -> Scope6/1
  Demux6/10 -> Terminator35/1
  Mux15/1 -> To Workspace1/1, State-Space10/1
  State-Space30/1 -> Mux15/1
  Demux4/4 -> Sum40/1, Sum36/1
  Demux6/9 -> Sum40/2, Goto19/1, Mux14/2
  Demux6/7 -> Mux12/2, Goto17/1, Sum38/1  "\\theta_1"
  Mux11/1 -> Scope5/1
  Sum34/1 -> State-Space31/1
  State-Space37/1 -> Non Linear System5/4(Y)
  Demux5/2 -> Mux12/1, Sum34/1  "\\theta_1_lin"
  Demux6/2 -> Terminator39/1  "y"
  State-Space32/1 -> Mux15/4
  Sum36/1 -> State-Space32/1
  Demux6/12 -> Terminator37/1
  Demux5/4 -> Mux14/1, Sum36/2  "\\theta_3_lin"
  Demux5/3 -> Sum35/2, Mux13/1  "\\theta_2_lin"
  State-Space31/1 -> Mux15/2
  State-Space10/1 -> To Workspace/1, Demux5/1
  Sum35/1 -> State-Space33/1
  From19/1 -> Scope11/3
  From12/1 -> Mux/1, Scope9/1
  From22/1 -> Scope10/3
  From20/1 -> Scope10/1
  From15/1 -> Scope12/3
  From16/1 -> Scope9/3, Mux/3
  From21/1 -> Scope10/2
  From17/1 -> Scope11/1
  From23/1 -> Scope12/1
  From14/1 -> Scope12/2
  From18/1 -> Scope11/2
  From13/1 -> Mux/2, Scope9/2
  Mux/1 -> To Workspace4/1
  Sum42/1 -> Mux16/2
  Demux16/4 -> Sum44/1
  Demux16/1 -> Sum41/2
  Demux17/1 -> Sum41/1, Scope13/1  "z_lin"
  Sum44/1 -> Mux16/4
  Sum43/1 -> Mux16/3
  Demux17/4 -> Sum44/2, Scope16/1  "\\theta_3_lin"
  State-Space/1 -> Demux17/1
  Demux17/2 -> Sum42/1, Scope14/1  "\\theta_1_lin"
  Sum41/1 -> Mux16/1
  Demux17/3 -> Scope15/1, Sum43/2  "\\theta_2_lin"
  Mux1/1 -> Demux19/1, Demux16/1, Demux1/1, Demux4/1, Demux9/1, Demux10/1, Demux13/1
  Demux16/2 -> Sum42/2
  Demux16/3 -> Sum43/1
  Mux16/1 -> State-Space/1
  Interpreted MATLAB Function1/1 -> Integrator1/1
  Mux17/1 -> Interpreted MATLAB Function1/1
  Mux19/1 -> Mux17/2
  Integrator1/1 -> Demux18/1, Mux17/1
  Demux19/3 -> Sum47/1
  Demux19/1 -> Sum45/2
  Demux19/2 -> Sum46/2
  Demux19/4 -> Sum48/1
  Demux18/3 -> Sum45/1, Scope17/1  "z"
  Demux18/7 -> Scope19/1, Sum46/1  "\\theta_1"
  Demux18/8 -> Scope20/1, Sum47/2  "\\theta_2"
  Demux18/9 -> Scope18/1, Sum48/2  "\\theta_3"
  Demux18/1 -> Terminator40/1  "x"
  Demux18/2 -> Terminator41/1  "y"
  Demux18/4 -> Terminator42/1
  Demux18/6 -> Terminator44/1
  Demux18/5 -> Terminator43/1
  Demux18/10 -> Terminator45/1
  Demux18/11 -> Terminator46/1
  Demux18/12 -> Terminator47/1
  [th2_PID] -> Scope20/2
  [z_PID] -> Scope17/2
  [th1_PID] -> Scope19/2
  [th3_PID] -> Scope18/2
  Sum45/1 -> MyPID/1(zd-z(t))
  MyPID/1(H) -> Mux19/1
  Sum48/1 -> MyPID4/1(In1)
  Sum47/1 -> MyPID2/1(In1)
  MyPID1/1(Out1) -> Mux19/2
  Sum46/1 -> MyPID1/1(In1)
  MyPID2/1(Out1) -> Mux19/3
  MyPID4/1(Out1) -> Mux19/4

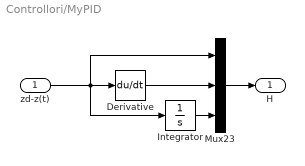
== system Controllori/MyPID ==
  zd-z(t) : Inport
  Derivative : Derivative
  Integrator : Integrator
  Mux23 : Mux  Inputs=3
  H : Outport
  wires:
  zd-z(t)/1 -> Integrator/1, Mux23/1, Derivative/1
  Derivative/1 -> Mux23/2
  Integrator/1 -> Mux23/3
  Mux23/1 -> H/1

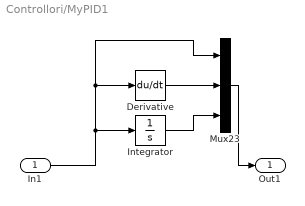
== system Controllori/MyPID1 ==
  In1 : Inport
  Derivative : Derivative
  Integrator : Integrator
  Mux23 : Mux  Inputs=3
  Out1 : Outport
  wires:
  In1/1 -> Mux23/1, Derivative/1, Integrator/1
  Derivative/1 -> Mux23/2
  Integrator/1 -> Mux23/3
  Mux23/1 -> Out1/1

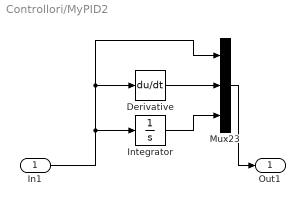
== system Controllori/MyPID2 ==
  In1 : Inport
  Derivative : Derivative
  Integrator : Integrator
  Mux23 : Mux  Inputs=3
  Out1 : Outport
  wires:
  In1/1 -> Mux23/1, Derivative/1, Integrator/1
  Derivative/1 -> Mux23/2
  Integrator/1 -> Mux23/3
  Mux23/1 -> Out1/1

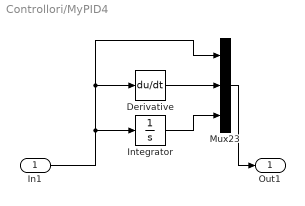
== system Controllori/MyPID4 ==
  In1 : Inport
  Derivative : Derivative
  Integrator : Integrator
  Mux23 : Mux  Inputs=3
  Out1 : Outport
  wires:
  In1/1 -> Mux23/1, Derivative/1, Integrator/1
  Derivative/1 -> Mux23/2
  Integrator/1 -> Mux23/3
  Mux23/1 -> Out1/1

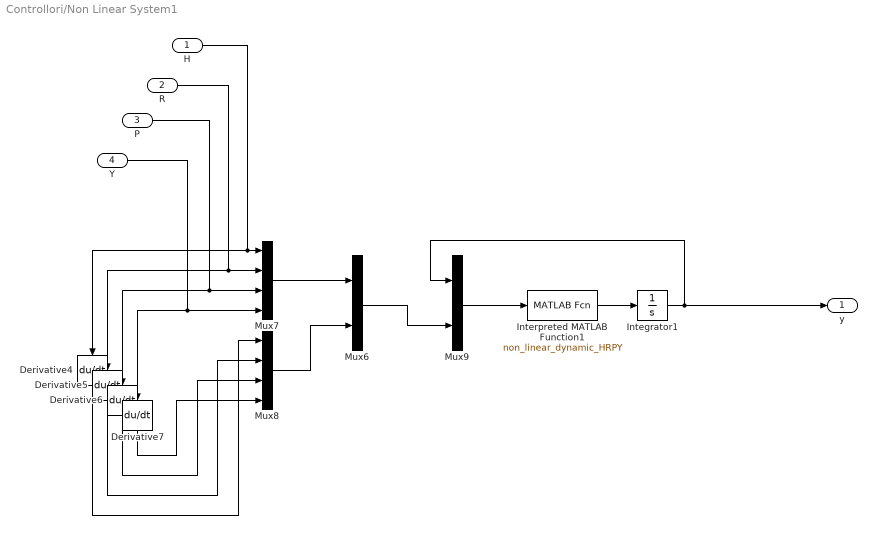
== system Controllori/Non Linear System1 ==
  H : Inport
  R : Inport  Port=2
  P : Inport  Port=3
  Y : Inport  Port=4
  Derivative{4..7} (4 alike) : Derivative
  Integrator1 : Integrator  InitialCondition=[0,0,0,0,0,0,0,0,0,0,0,0]
  Interpreted MATLAB Function1 : MATLABFcn  MATLABFcn=non_linear_dynamic_HRPY
  Mux6 : Mux  Inputs=2
  Mux7 : Mux
  Mux8 : Mux
  Mux9 : Mux  Inputs=2
  y : Outport
  wires:
  Integrator1/1 -> y/1, Mux9/1
  Mux6/1 -> Mux9/2
  H/1 -> Derivative4/1, Mux7/1
  Mux7/1 -> Mux6/1
  R/1 -> Derivative5/1, Mux7/2
  Mux8/1 -> Mux6/2
  P/1 -> Mux7/3, Derivative6/1
  Interpreted MATLAB Function1/1 -> Integrator1/1
  Derivative7/1 -> Mux8/4
  Derivative4/1 -> Mux8/1
  Mux9/1 -> Interpreted MATLAB Function1/1
  Y/1 -> Mux7/4, Derivative7/1
  Derivative5/1 -> Mux8/2
  Derivative6/1 -> Mux8/3

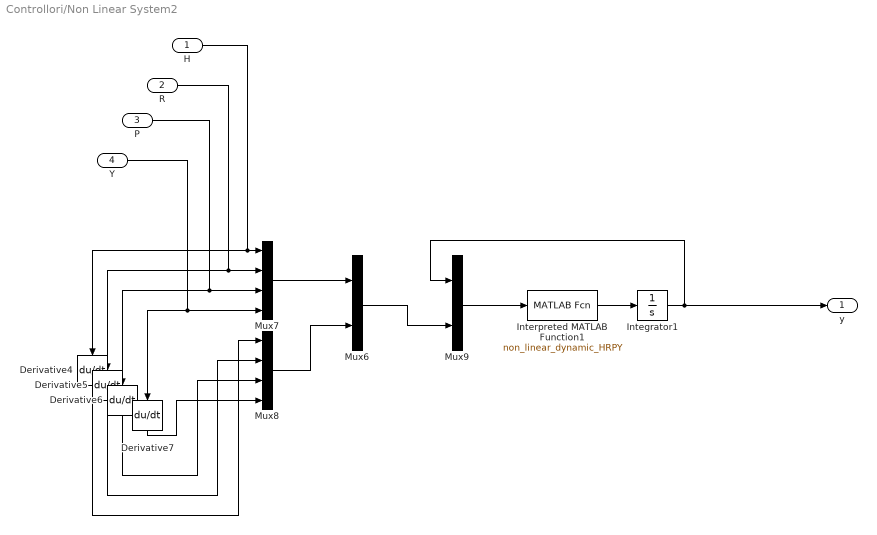
== system Controllori/Non Linear System2 ==
  H : Inport
  R : Inport  Port=2
  P : Inport  Port=3
  Y : Inport  Port=4
  Derivative{4..7} (4 alike) : Derivative
  Integrator1 : Integrator  InitialCondition=[0,0,0,0,0,0,0,0,0,0,0,0]
  Interpreted MATLAB Function1 : MATLABFcn  MATLABFcn=non_linear_dynamic_HRPY
  Mux6 : Mux  Inputs=2
  Mux7 : Mux
  Mux8 : Mux
  Mux9 : Mux  Inputs=2
  y : Outport
  wires:
  Integrator1/1 -> y/1, Mux9/1
  Mux6/1 -> Mux9/2
  H/1 -> Derivative4/1, Mux7/1
  Mux7/1 -> Mux6/1
  R/1 -> Derivative5/1, Mux7/2
  Mux8/1 -> Mux6/2
  P/1 -> Mux7/3, Derivative6/1
  Interpreted MATLAB Function1/1 -> Integrator1/1
  Derivative7/1 -> Mux8/4
  Derivative4/1 -> Mux8/1
  Mux9/1 -> Interpreted MATLAB Function1/1
  Y/1 -> Mux7/4, Derivative7/1
  Derivative5/1 -> Mux8/2
  Derivative6/1 -> Mux8/3

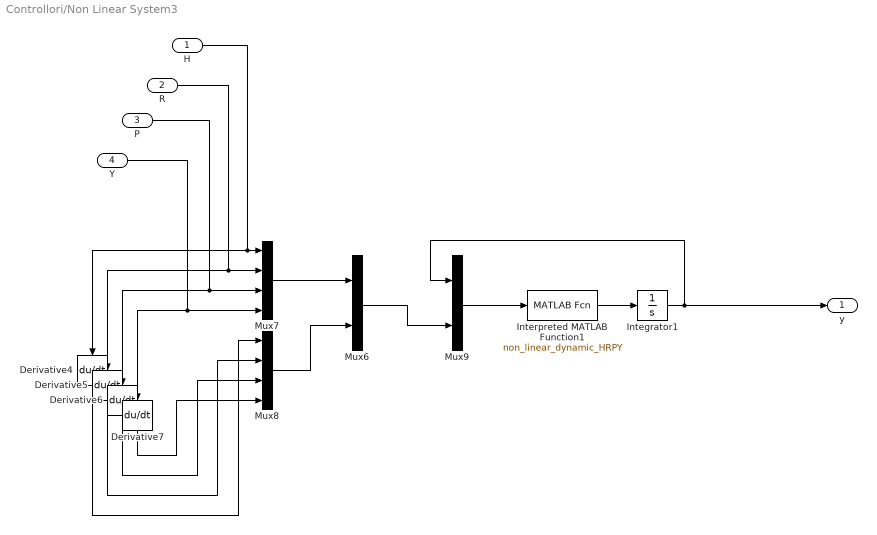
== system Controllori/Non Linear System3 ==
  H : Inport
  R : Inport  Port=2
  P : Inport  Port=3
  Y : Inport  Port=4
  Derivative{4..7} (4 alike) : Derivative
  Integrator1 : Integrator  InitialCondition=[0,0,0,0,0,0,0,0,0,0,0,0]
  Interpreted MATLAB Function1 : MATLABFcn  MATLABFcn=non_linear_dynamic_HRPY
  Mux6 : Mux  Inputs=2
  Mux7 : Mux
  Mux8 : Mux
  Mux9 : Mux  Inputs=2
  y : Outport
  wires:
  Integrator1/1 -> y/1, Mux9/1
  Mux6/1 -> Mux9/2
  H/1 -> Derivative4/1, Mux7/1
  Mux7/1 -> Mux6/1
  R/1 -> Derivative5/1, Mux7/2
  Mux8/1 -> Mux6/2
  P/1 -> Mux7/3, Derivative6/1
  Interpreted MATLAB Function1/1 -> Integrator1/1
  Derivative7/1 -> Mux8/4
  Derivative4/1 -> Mux8/1
  Mux9/1 -> Interpreted MATLAB Function1/1
  Y/1 -> Mux7/4, Derivative7/1
  Derivative5/1 -> Mux8/2
  Derivative6/1 -> Mux8/3

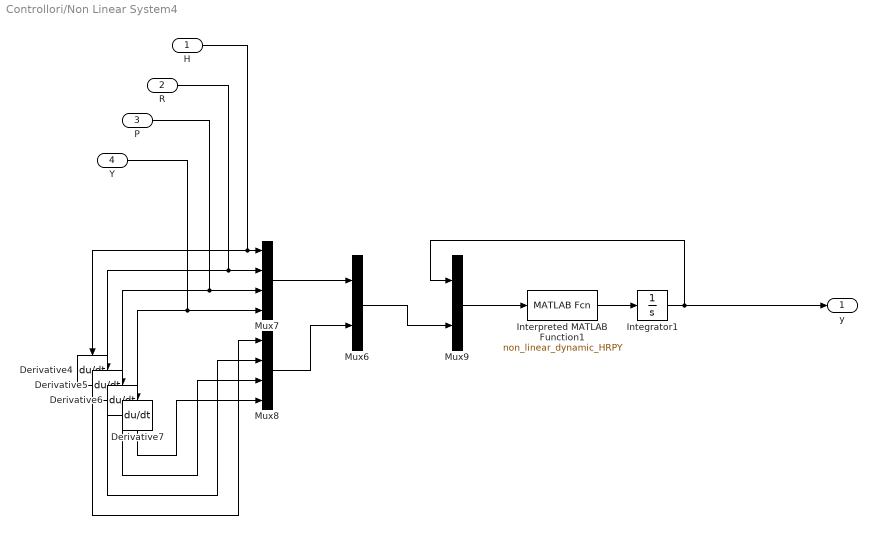
== system Controllori/Non Linear System4 ==
  H : Inport
  R : Inport  Port=2
  P : Inport  Port=3
  Y : Inport  Port=4
  Derivative{4..7} (4 alike) : Derivative
  Integrator1 : Integrator  InitialCondition=[0,0,0,0,0,0,0,0,0,0,0,0]
  Interpreted MATLAB Function1 : MATLABFcn  MATLABFcn=non_linear_dynamic_HRPY
  Mux6 : Mux  Inputs=2
  Mux7 : Mux
  Mux8 : Mux
  Mux9 : Mux  Inputs=2
  y : Outport
  wires:
  Integrator1/1 -> y/1, Mux9/1
  Mux6/1 -> Mux9/2
  H/1 -> Derivative4/1, Mux7/1
  Mux7/1 -> Mux6/1
  R/1 -> Derivative5/1, Mux7/2
  Mux8/1 -> Mux6/2
  P/1 -> Mux7/3, Derivative6/1
  Interpreted MATLAB Function1/1 -> Integrator1/1
  Derivative7/1 -> Mux8/4
  Derivative4/1 -> Mux8/1
  Mux9/1 -> Interpreted MATLAB Function1/1
  Y/1 -> Mux7/4, Derivative7/1
  Derivative5/1 -> Mux8/2
  Derivative6/1 -> Mux8/3

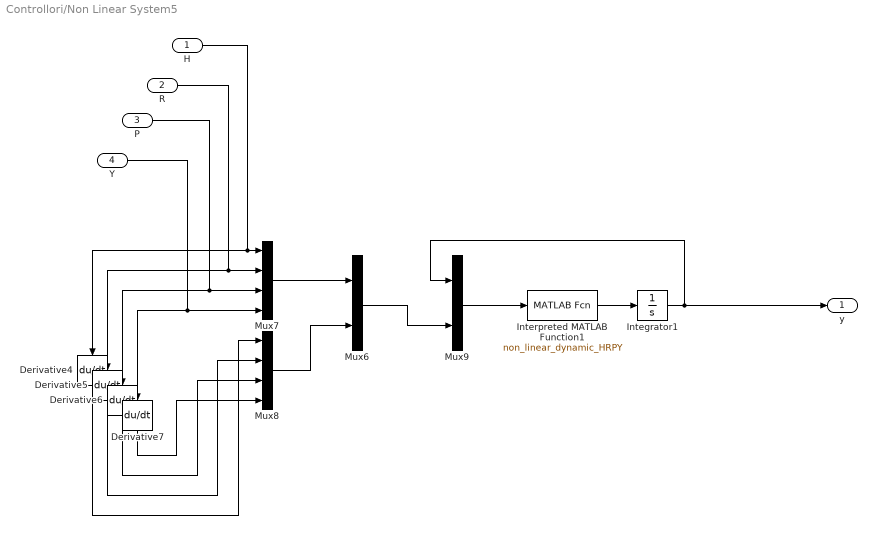
== system Controllori/Non Linear System5 ==
  H : Inport
  R : Inport  Port=2
  P : Inport  Port=3
  Y : Inport  Port=4
  Derivative{4..7} (4 alike) : Derivative
  Integrator1 : Integrator  InitialCondition=[0,0,0,0,0,0,0,0,0,0,0,0]
  Interpreted MATLAB Function1 : MATLABFcn  MATLABFcn=non_linear_dynamic_HRPY
  Mux6 : Mux  Inputs=2
  Mux7 : Mux
  Mux8 : Mux
  Mux9 : Mux  Inputs=2
  y : Outport
  wires:
  Integrator1/1 -> y/1, Mux9/1
  Mux6/1 -> Mux9/2
  H/1 -> Derivative4/1, Mux7/1
  Mux7/1 -> Mux6/1
  R/1 -> Derivative5/1, Mux7/2
  Mux8/1 -> Mux6/2
  P/1 -> Mux7/3, Derivative6/1
  Interpreted MATLAB Function1/1 -> Integrator1/1
  Derivative7/1 -> Mux8/4
  Derivative4/1 -> Mux8/1
  Mux9/1 -> Interpreted MATLAB Function1/1
  Y/1 -> Mux7/4, Derivative7/1
  Derivative5/1 -> Mux8/2
  Derivative6/1 -> Mux8/3
